simulink model "WindTurbine_System"  (R2023b)
settings: Solver=FixedStepAuto  StartTime=0.0  StopTime=24  FixedStep=1e-6  MaxStep=1e-6  RelTol=1e-3
values from neighbouring files (symbols this model uses):
  c1 = 0.22    [SystemParams.m]    (also in WindTurbineScript.m)
  c2 = 116    [SystemParams.m]    (also in WindTurbineScript.m)
  c3 = 0.4    [SystemParams.m]    (also in WindTurbineScript.m)
  c5 = 5    [SystemParams.m]    (also in WindTurbineScript.m)
  c6 = 12.5    [SystemParams.m]    (also in WindTurbineScript.m)
  C_boost = 50e-6    (= 5e-05)    [SystemParams.m]
  C_buck = 5e-6    (= 5e-06)    [SystemParams.m]
  C_rectifier = 1e-3    (= 0.001)    [SystemParams.m]
  Cp_sys = (Nr_cells_parallel * Cp_cell) / Nr_cells_series    [SystemParams.m]    (also in baterie.m)
  J = 0.8e-3    (= 0.0008)    [SystemParams.m]
  Ke = 0.175    [SystemParams.m]
  L_boost = 200e-6    (= 0.0002)    [SystemParams.m]
  L_buck = 300e-6    (= 0.0003)    [SystemParams.m]
  lambda_opt = 6.33    [SystemParams.m]    (also in WindTurbineScript.m)
  Ld = 1.53e-3    (= 0.00153)    [SystemParams.m]
  Lq = 1.53e-3    (= 0.00153)    [SystemParams.m]
  n1 = 15    [SystemParams.m]
  n2 = 1000    [SystemParams.m]
  omega_r = lambda_opt * wind_speed / R    (= 15.192)    [SystemParams.m]    (also in WindTurbineScript.m = omega_r_values(i))
  p = 4    [SystemParams.m]
  P_buck_v = 1.0e+03 * [0.01, 0.0427, 0.0854, 0.1282, 0.1709, 0.2136, 0.2563, 0.2990, 0.3418, 0.3845, 0.4272,                        0.4699, 0.5126, 0.5554, 0.5981, 0.6408, 0.6835, 0.7262, 0.7690, 0.8117, 0.8544,                        0.8971, 0.9398, 0.9826, 1.0253, 1.0680, 1.1107, 1.1534, 1.1962, 1.2389, 1.2816,                        1.3243, 1.3670, 1.4098, 1.4525, 1.4952, 1.5379, 1.5806, 1.6234, 1.6661, 1. ...(+623 chars)    [SystemParams.m]
  P_rec_v = 1.0e+03 * [0.01, 0.0432, 0.0864, 0.1296, 0.1727, 0.2159, 0.2591, 0.3023, 0.3455, 0.3887, 0.4319,                      0.4750, 0.5182, 0.5614, 0.6046, 0.6478, 0.6910, 0.7342, 0.7773, 0.8205, 0.8637,                      0.9069, 0.9501, 0.9933, 1.0365, 1.0796, 1.1228, 1.1660, 1.2092, 1.2524, 1.2956,                      1.3388, 1.3820, 1.4251, 1.4683, 1.5115, 1.5547, 1.5979, 1.6411, 1.6843, 1.7274,  ...(+605 chars)    [SystemParams.m]
  R = 5    [SystemParams.m]    (also in WindTurbineScript.m)
  R_buck_load_v = [230.4000, 53.9326, 26.9663, 17.9775, 13.4831, 10.7865, 8.9888, 7.7047, 6.7416, 5.9925, 5.3933,                   4.9030, 4.4944, 4.1487, 3.8523, 3.5955, 3.3708, 3.1725, 2.9963, 2.8386, 2.6966, 2.5682,                   2.4515, 2.3449, 2.2472, 2.1573, 2.0743, 1.9975, 1.9262, 1.8597, 1.7978, 1.7398, 1.6854,                   1.6343, 1.5863, 1.5409, 1.4981, 1.4576, 1.4193, 1.3829, 1.3483, 1.3154, 1. ...(+577 chars)    [SystemParams.m]
  R_rec_load_v = 1.0e+03 * [4.8400, 1.1204, 0.5602, 0.3735, 0.2803, 0.2242, 0.1868, 0.1601, 0.1401, 0.1245, 0.1121,                            0.1019, 0.0934, 0.0862, 0.0801, 0.0747, 0.0700, 0.0659, 0.0623, 0.0590, 0.0560, 0.0534,                            0.0509, 0.0487, 0.0467, 0.0448, 0.0431, 0.0415, 0.0400, 0.0386, 0.0374, 0.0362, 0.0350,                            0.0340, 0.0330, 0.0320, 0.0311, 0.0303, 0.02 ...(+634 chars)    [SystemParams.m]
  ro = 1.225    [SystemParams.m]    (also in WindTurbineScript.m)
  Rp_sys = (Nr_cells_series * Rp_cell) / Nr_cells_parallel    [SystemParams.m]    (also in baterie.m)
  Rs = 2.875    [SystemParams.m]    (also in VOC_1C_3pulse_14rest.mat = 0.09415625)
  Rs_sys = (Nr_cells_series * Rs_cell) / Nr_cells_parallel    [SystemParams.m]    (also in baterie.m)
  State_Of_Charge = 65    [SystemParams.m]
libraries: simulink x4, slpidlib x2, SignalEditorBlockLib x1
(part 1 of 2)
settings Model: SimulationMode=accelerator  Creator=tudorn  LastModifiedBy=tudorn
settings HardwareCC: ProdBitPerLong=64  ProdHWDeviceType=Apple->ARM64

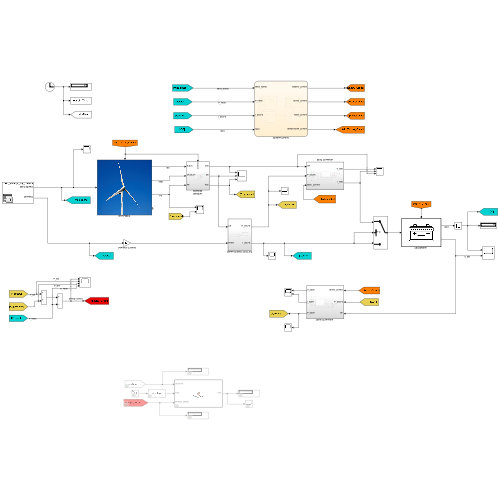
[thumbnail: Simulink's stored preview of the top-level diagram]
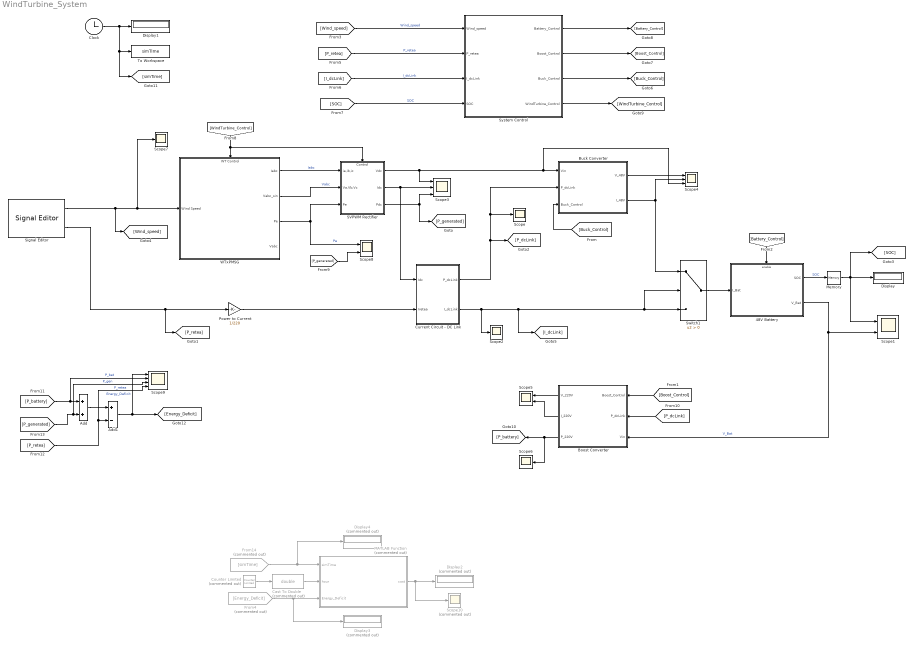
== system WindTurbine_System ==
  "48V Battery " : Subsystem
      mask Display: image('batteryPhoto.png');
  Add : Sum
  Add1 : Sum  Inputs=+-
  Boost Converter : Subsystem
  Buck Converter : Subsystem
  Cast To Double : DataTypeConversion  Commented=on  OutDataTypeStr=double  SaturateOnIntegerOverflow=off  RndMeth=Floor
  Clock : Clock
  Counter Limited : simulink/Sources/Counter Limited  Commented=on  uplimit=24  tsamp=1
  Current Circuit - DC Link : Subsystem
  Display : Display
  Display1 : Display
  Display2 : Display  Commented=on
  Display3 : Display  Commented=on
  Display4 : Display  Commented=on
  From14 : From  Commented=on  GotoTag=simTime
  From4 : From  Commented=on  GotoTag=Energy_Deficit
  MATLAB Function : MATLAB Function  Commented=on  TreatAsAtomicUnit=on
  Memory : Memory  InitialCondition=State_Of_Charge
  Power to Current : Gain  Gain=1/220
  SVPWM Rectifier : Subsystem
      settings: PortSchema="{\"entries\":[{\"content\":{\"sides\":[{\"content\":{\"connectorIds\":[\"In1\",\"In2\",\"In3\"]},\"type\":\"ConnectorPlacement.EquallySpacedRectSide\",\"uuid\":\"47eca95a-203c-4150-b63f-06b4ee16708d\"},{\"content\":{\"connectorIds\":[\"Out1\",\"Out2\",\"Out3\"],\"side\":\"RIGHT\"},\"type\":\"ConnectorPlacement.EquallySpacedRectSide\",\"uuid\":\"e6ad715a-a702-4d71-ac1c-337baa4d9820\"},{\"content\":{\"connectorIds\":[\"In4\"],\"side\":\"TOP\"},\"type\":\"ConnectorPlacement.EquallySpacedRectSide\",\"uuid\":\"da1a96bd-35b5-4cd5-85b2-7e6a1b4649ba\"}]},\"type\":\"ConnectorPlacement.EquallySpacedConnector\",\"uuid\":\"95ca3103-3ae0-40eb-bfd8-7b543be5b023\"}],\"packageUris\":[\"http://schema.mathworks.com/mf0/Connector/R2020b\"],\"version\":\"1.0\"}"
  Scope{,2,6..7} (4 alike) : Scope
  Scope1 : Scope  NumInputPorts=2
  Scope10 : Scope  Commented=on
  Scope3 : Scope  NumInputPorts=3
  Scope4 : Scope  NumInputPorts=3
  Scope5 : Scope  NumInputPorts=2
  Scope8 : Scope  NumInputPorts=2
  Scope9 : Scope  NumInputPorts=4
  Signal Editor : SignalEditorBlockLib/Signal Editor  FileName=ConstWind_VarDemand.mat  ActiveScenario=x24h_Increase_WS_Demand  ActiveSignal=Wind Speed  IsBus=off  OutputBusObjectStr=Bus: BusObject  SampleTime=0  Interpolate=off  ZeroCross=off  OutputAfterFinalValue=Setting to zero  Unit=inherit  PreserveSignalName=on  ApplySigPropsToAllScenarios=on  ApplySigPropsToAllSignals=off
  Switch1 : Switch  Criteria=u2 > Threshold  SaturateOnIntegerOverflow=off  InputSameDT=off
  System Control : Stateflow chart  TreatAsAtomicUnit=on
  To Workspace : ToWorkspace  VariableName=simTIme  SaveFormat=Timeseries  SampleTime=-1
  WTxPMSG : Subsystem
      settings: PortSchema="{\"entries\":[{\"content\":{\"sides\":[{\"content\":{\"connectorIds\":[\"In1\"]},\"type\":\"ConnectorPlacement.EquallySpacedRectSide\",\"uuid\":\"6e920366-051d-4787-8dda-26163d9164f0\"},{\"content\":{\"connectorIds\":[\"Out1\",\"Out2\",\"Out3\",\"Out4\"],\"side\":\"RIGHT\"},\"type\":\"ConnectorPlacement.EquallySpacedRectSide\",\"uuid\":\"50211027-c95a-4b04-b652-faaace106a3a\"},{\"content\":{\"connectorIds\":[\"In2\"],\"side\":\"TOP\"},\"type\":\"ConnectorPlacement.EquallySpacedRectSide\",\"uuid\":\"d93d5085-7e12-4e15-83b4-3ac4d8b1a417\"}]},\"type\":\"ConnectorPlacement.EquallySpacedConnector\",\"uuid\":\"325f5742-bcf0-41bb-9a35-ab4334df2944\"}],\"packageUris\":[\"http://schema.mathworks.com/mf0/Connector/R2020b\"],\"version\":\"1.0\"}"
      mask Display: image('windTurbinePhoto.png');
  wires:
  [P_generated] -> Scope9/3, Add/2  "P_gen"
  WTxPMSG/3(Pe) -> SVPWM Rectifier/3(Pe), Scope8/1  "Pe"
  "48V Battery "/2(V_Bat) -> Boost Converter/3(Vin), Scope1/2  "V_Bat"
  [Buck_Control] -> Buck Converter/3(Buck_Control)
  [WindTurbine_Control] -> SVPWM Rectifier/4(Control), WTxPMSG/2(WT Control)
  Current Circuit - DC Link/2(I_dcLink) -> Scope2/1, [I_dcLink], Switch1/2, Switch1/3
  Current Circuit - DC Link/1(P_dcLink) -> [P_dcLink], Scope/1, Buck Converter/2(P_dcLink)
  [P_battery] -> Scope9/2, Add/1  "P_bat"
  Boost Converter/1(V_220V) -> Scope5/1
  Add/1 -> Add1/1
  Power to Current/1 -> Current Circuit - DC Link/2(Iretea)
  WTxPMSG/2(Vabc_sin) -> SVPWM Rectifier/2(Va,Vb,Vc)  "Vabc"
  Switch1/1 -> "48V Battery "/1(I_Bat)
  "48V Battery "/1(SOC) -> Memory/1  "SOC"
  Buck Converter/2(I_48V) -> Scope4/2, Switch1/1
  SVPWM Rectifier/3(Pdc) -> Scope3/3, [P_generated]
  [Battery_Control] -> "48V Battery "/Enable
  Buck Converter/1(V_48V) -> Scope4/1
  [P_dcLink] -> Boost Converter/2(P_dcLink)
  Memory/1 -> [SOC], Display/1, Scope1/1
  [P_generated] -> Scope8/2
  SVPWM Rectifier/1(Vdc) -> Scope4/3, Buck Converter/1(Vin), Scope3/1
  WTxPMSG/1(Iabc) -> SVPWM Rectifier/1(ia,ib,ic)  "Iabc"
  Signal Editor/1 -> Scope7/1, WTxPMSG/1(Wind Speed), [Wind_speed]
  Signal Editor/2 -> Power to Current/1, [P_retea]
  Clock/1 -> [simTime], To Workspace/1, Display1/1
  [P_retea] -> Scope9/4, Add1/2  "P_retea"
  Boost Converter/2(I_220V) -> Scope5/2
  Add1/1 -> Scope9/1, [Energy_Deficit]  "Energy_Deficit"
  [Boost_Control] -> Boost Converter/1(Boost_Control)
  Boost Converter/3(P_220V) -> [P_battery], Scope6/1
  SVPWM Rectifier/2(Idc) -> Scope3/2, Current Circuit - DC Link/1(Idc)
  [P_retea] -> System Control/2(P_retea)  "P_retea"
  [Wind_speed] -> System Control/1(Wind_speed)  "Wind_speed"
  System Control/3(Buck_Control) -> [Buck_Control]
  [I_dcLink] -> System Control/3(I_dcLink)  "I_dcLink"
  System Control/4(WindTurbine_Control) -> [WindTurbine_Control]
  [SOC] -> System Control/4(SOC)  "SOC"
  System Control/2(Boost_Control) -> [Boost_Control]
  System Control/1(Battery_Control) -> [Battery_Control]
  MATLAB Function/1(cost) -> Scope10/1, Display2/1
  From4/1 -> Display3/1, MATLAB Function/3(Energy_Deficit)
  From14/1 -> Display4/1, MATLAB Function/1(simTime)
  Counter Limited/1 -> Cast To Double/1
  Cast To Double/1 -> MATLAB Function/2(hour)

== system WindTurbine_System/48V Battery  ==
  I_Bat : Inport
  Enable : EnablePort
  (14 - 96)% SOC : Saturate  UpperLimit=96  LowerLimit=14
  Add : Sum  Inputs=+++
  Cp : Constant  Value=Cp_sys
  RC Network : Subsystem
  Rp : Constant  Value=Rp_sys
  Rs : Gain  Gain=Rs_sys
  SOC Calculation1 : Subsystem
  SOC_OCV : Subsystem
  Saturation : Saturate  UpperLimit=93.75  LowerLimit=-93.75
  Scope : Scope
  Scope1 : Scope
  Scope2 : Scope
  SOC : Outport
  V_Bat : Outport  Port=2
  wires:
  RC Network/1(V1) -> Scope2/1, Add/2
  SOC_OCV/1(OCV) -> Add/1
  Rp/1 -> RC Network/2(Rp)
  Cp/1 -> RC Network/3(Cp)
  Rs/1 -> Add/3  "Vs - Voltage drop on the Series Resistance"
  Add/1 -> Scope1/1, V_Bat/1
  SOC Calculation1/1(SOC) -> (14 - 96)% SOC/1
  (14 - 96)% SOC/1 -> Scope/1, SOC/1, SOC_OCV/1(SOC)
  I_Bat/1 -> Saturation/1
  Saturation/1 -> SOC Calculation1/1(I_Bat), Rs/1, RC Network/1(I_Bat)

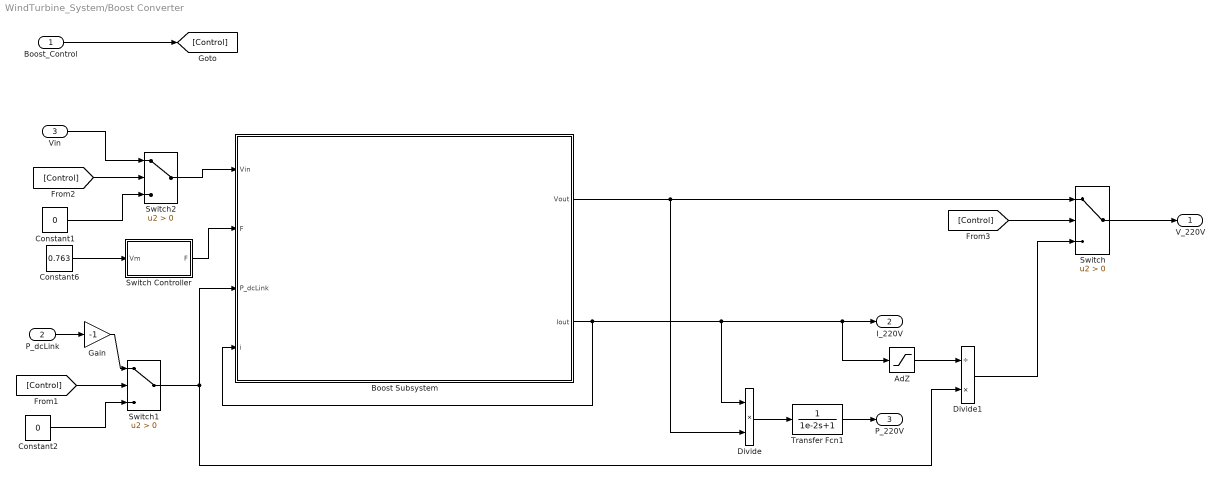
== system WindTurbine_System/Boost Converter ==
  Boost_Control : Inport
  P_dcLink : Inport  Port=2
  Vin : Inport  Port=3
  AdZ : Saturate  UpperLimit=inf  LowerLimit=1e-6
  Boost Subsystem : Subsystem
  Constant1 : Constant  Value=0
  Constant2 : Constant  Value=0
  Constant6 : Constant  Value=0.763
  Divide : Product  Inputs=**
  Divide1 : Product  Inputs=/*
  Gain : Gain  Gain=-1
  Switch : Switch  Criteria=u2 > Threshold  SaturateOnIntegerOverflow=off  InputSameDT=off
  Switch Controller : Subsystem
  Switch1 : Switch  Criteria=u2 > Threshold  SaturateOnIntegerOverflow=off  InputSameDT=off
  Switch2 : Switch  Criteria=u2 > Threshold  SaturateOnIntegerOverflow=off  InputSameDT=off
  Transfer Fcn1 : TransferFcn  Denominator=[1e-2 1]
  V_220V : Outport
  I_220V : Outport  Port=2
  P_220V : Outport  Port=3
  wires:
  Constant6/1 -> Switch Controller/1(Vm)
  Switch Controller/1(F) -> Boost Subsystem/2(F)
  Divide/1 -> Transfer Fcn1/1
  Transfer Fcn1/1 -> P_220V/1
  Boost Subsystem/1(Vout) -> Switch/1, Divide/2
  Boost Subsystem/2(Iout) -> Divide/1, AdZ/1, I_220V/1, Boost Subsystem/4(i)
  Boost_Control/1 -> [Control]
  Constant1/1 -> Switch2/3
  [Control] -> Switch2/2
  Switch2/1 -> Boost Subsystem/1(Vin)
  Vin/1 -> Switch2/1
  Constant2/1 -> Switch1/3
  [Control] -> Switch1/2
  P_dcLink/1 -> Gain/1
  Gain/1 -> Switch1/1
  Switch1/1 -> Divide1/2, Boost Subsystem/3(P_dcLink)
  [Control] -> Switch/2
  Switch/1 -> V_220V/1
  Divide1/1 -> Switch/3
  AdZ/1 -> Divide1/1

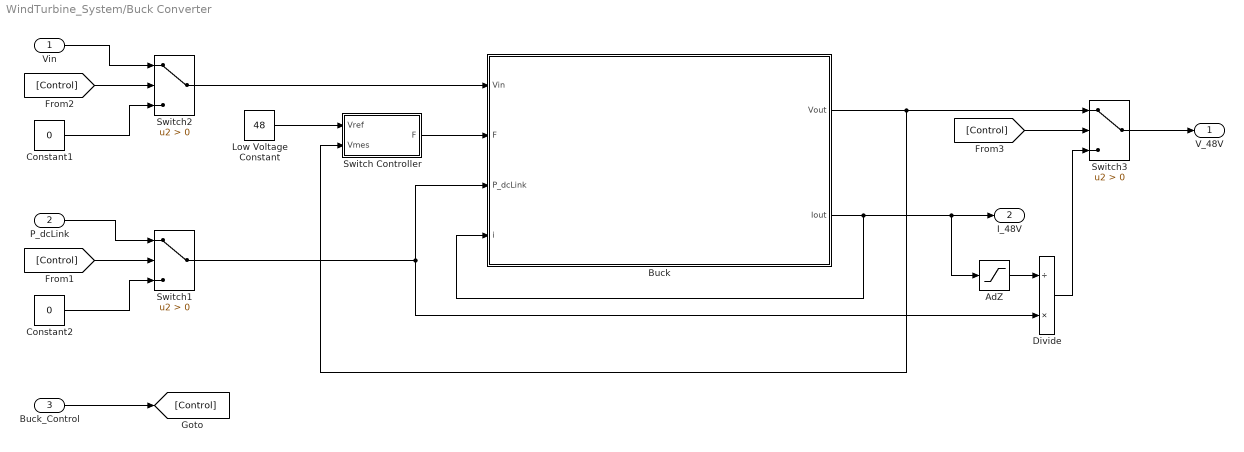
== system WindTurbine_System/Buck Converter ==
  Vin : Inport
  P_dcLink : Inport  Port=2
  Buck_Control : Inport  Port=3
  AdZ : Saturate  UpperLimit=inf  LowerLimit=1e-6
  Buck : Subsystem
  Constant1 : Constant  Value=0
  Constant2 : Constant  Value=0
  Divide : Product  Inputs=/*
  Low Voltage Constant : Constant  Value=48
  Switch Controller : Subsystem
  Switch1 : Switch  Criteria=u2 > Threshold  SaturateOnIntegerOverflow=off  InputSameDT=off
  Switch2 : Switch  Criteria=u2 > Threshold  SaturateOnIntegerOverflow=off  InputSameDT=off
  Switch3 : Switch  Criteria=u2 > Threshold  SaturateOnIntegerOverflow=off  InputSameDT=off
  V_48V : Outport
  I_48V : Outport  Port=2
  wires:
  Low Voltage Constant/1 -> Switch Controller/1(Vref)
  Switch Controller/1(F) -> Buck/2(F)
  Buck/1(Vout) -> Switch Controller/2(Vmes), Switch3/1
  Buck/2(Iout) -> AdZ/1, I_48V/1, Buck/4(i)
  Buck_Control/1 -> [Control]
  [Control] -> Switch2/2
  Constant1/1 -> Switch2/3
  Switch2/1 -> Buck/1(Vin)
  Vin/1 -> Switch2/1
  Constant2/1 -> Switch1/3
  [Control] -> Switch1/2
  Switch1/1 -> Divide/2, Buck/3(P_dcLink)
  P_dcLink/1 -> Switch1/1
  Switch3/1 -> V_48V/1
  [Control] -> Switch3/2
  Divide/1 -> Switch3/3
  AdZ/1 -> Divide/1

== system WindTurbine_System/Current Circuit - DC Link ==
  Idc : Inport
  Iretea : Inport  Port=2
  Add : Sum  Inputs=+-
  Gain : Gain  Gain=220
  P_dcLink : Outport
  I_dcLink : Outport  Port=2
  wires:
  Idc/1 -> Add/1
  Iretea/1 -> Add/2
  Add/1 -> Gain/1, I_dcLink/1
  Gain/1 -> P_dcLink/1

== system WindTurbine_System/SVPWM Rectifier ==
  ia,ib,ic : Inport
  Va,Vb,Vc : Inport  Port=2
  Pe : Inport  Port=3
  Control : Inport  Port=4
  AdZ : Saturate  UpperLimit=inf  LowerLimit=1e-6
  Divide : Product  Inputs=**
  Divide1 : Product  Inputs=/*
  Saturation : Saturate  UpperLimit=220  LowerLimit=0
  Space Vector PWM : Subsystem
  Switch : Switch  Criteria=u2 > Threshold  SaturateOnIntegerOverflow=off  InputSameDT=off
  V_DC Calculation : Subsystem
  Vdc : Outport
  Idc : Outport  Port=2
  Pdc : Outport  Port=3
  wires:
  Va,Vb,Vc/1 -> Space Vector PWM/1("Va, Vb, Vc")
  V_DC Calculation/2(Idc) -> AdZ/1, Idc/1, Divide/1
  ia,ib,ic/1 -> V_DC Calculation/1("Ia, Ib, Ic")
  Space Vector PWM/1(Sa,Sb,Sc) -> V_DC Calculation/2("Sa, Sb, Sc")
  Pe/1 -> V_DC Calculation/3(Pe), Divide1/2
  Switch/1 -> Vdc/1
  Control/1 -> Switch/2
  V_DC Calculation/1(Vdc) -> Switch/1, Divide/2
  Divide1/1 -> Saturation/1
  Divide/1 -> Pdc/1
  AdZ/1 -> Divide1/1
  Saturation/1 -> Switch/3

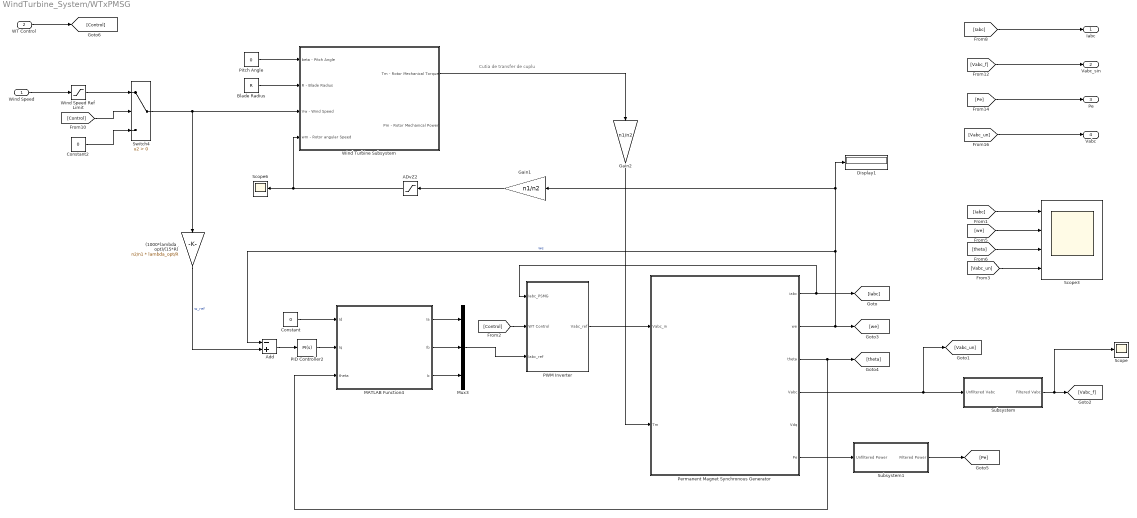
== system WindTurbine_System/WTxPMSG ==
  note: Cutia de transfer de cuplu
  Wind Speed : Inport
  WT Control : Inport  Port=2
  (1000*lambda_opt)/(15*R) : Gain  Gain=n2/n1 * lambda_opt/R
  ADvZ2 : Saturate  UpperLimit=omega_r  LowerLimit=1e-6
  Add : Sum  Inputs=-+
  Blade Radius : Constant  Value=R
  Constant : Constant  Value=0
  Constant2 : Constant  Value=0
  Display1 : Display
  Gain1 : Gain  Gain=n1/n2
  Gain2 : Gain  Gain=n1/n2
  MATLAB Function4 : MATLAB Function  TreatAsAtomicUnit=on
  Mux3 : Mux  Inputs=3
  PID Controller2 : slpidlib/PID Controller  Controller=PI  Form=Parallel  TimeDomain=Continuous-time  UseExternalTs=off  SampleTime=-1  IntegratorMethod=Forward Euler  FilterMethod=Forward Euler  ControllerParametersSource=internal  P=40  I=3  UseKiTs=off  D=0  N=100  UseFilter=on  TunerSelectOption=Transfer Function Based (PID Tuner App)  InitialConditionSource=internal  InitialConditionForIntegrator=0  InitialConditionForFilter=0  DifferentiatorICPrevScaledInput=0  ExternalReset=none  TrackingMode=off  Kt=1  LimitOutput=off  SatLimitsSource=internal  UpperSaturationLimit=inf  LowerSaturationLimit=-inf  LinearizeAsGain=on  AntiWindupMode=none  Kb=1  LimitIntegrator=off  UpperIntegratorSaturationLimit=inf  LowerIntegratorSaturationLimit=-inf  POutMin=[]  POutMax=[]  IOutMin=[]  IOutMax=[]  DOutMin=[]  DOutMax=[]  NOutMin=[]  NOutMax=[]  SumOutMin=[]  SumOutMax=[]  SaturationOutMin=[]  SaturationOutMax=[]  PParamMin=[]  PParamMax=[]  IParamMin=[]  IParamMax=[]  DParamMin=[]  DParamMax=[]  NParamMin=[]  NParamMax=[]  KbParamMin=[]  KbParamMax=[]  KtParamMin=[]  KtParamMax=[]  KbOutMin=[]  KbOutMax=[]  KtOutMin=[]  KtOutMax=[]  IntegratorOutMin=[]  IntegratorOutMax=[]  FilterOutMin=[]  FilterOutMax=[]  SumI1OutMin=[]  SumI1OutMax=[]  SumI2OutMin=[]  SumI2OutMax=[]  SumI3OutMin=[]  SumI3OutMax=[]  SumI4OutMin=[]  SumI4OutMax=[]  SumDOutMin=[]  SumDOutMax=[]  DifferentiatorOutMin=[]  DifferentiatorOutMax=[]  FilterDiffOutCoefMin=[]  FilterDiffOutCoefMax=[]  ReciprocalOutMin=[]  ReciprocalOutMax=[]  SumDenOutMin=[]  SumDenOutMax=[]  SumNumOutMin=[]  SumNumOutMax=[]  DivideOutMin=[]  DivideOutMax=[]  UdiffTsProdOutMin=[]  UdiffTsProdOutMax=[]  NTsProdOutMin=[]  NTsProdOutMax=[]  UintegralTsProdOutMin=[]  UintegralTsProdOutMax=[]  UngainTsProdOutMin=[]  UngainTsProdOutMax=[]  ClampingZeroOutDataTypeStr=Inherit: Inherit via back propagation  ClampingZeroOutMin=[]  ClampingZeroOutMax=[]  FilterDenConstantOutDataTypeStr=Inherit: Inherit via back propagation  FilterDenConstantOutMin=[]  FilterDenConstantOutMax=[]  PCopyOutDataTypeStr=Inherit: Inherit via back propagation  PCopyOutMin=[]  PCopyOutMax=[]  NCopyOutDataTypeStr=Inherit: Inherit via back propagation  NCopyOutMin=[]  NCopyOutMax=[]  IntegratorContinuousStateAttributes=''  IntegratorStateMustResolveToSignalObject=off  IntegratorRTWStateStorageClass=Auto  FilterContinuousStateAttributes=''  FilterStateMustResolveToSignalObject=off  FilterRTWStateStorageClass=Auto  ParallelPVariant=InternalParameters  IdealPVariant=Disabled  IVariant=InternalParameters  DVariant=Disabled  IntegratorVariant=Continuous  SatVariant=Disabled  AWVariant=Passthrough  PCopyVariant=Disabled  TRVariant=Disabled  FdbkBlocksVariant=Forward  IdealPFdbkVariant=Disabled  SatFdbkVariant=Disabled  DerivativeFilterVariant=Disabled  NVariant=Disabled  NCopyVariant=Disabled_SignalSpec  FilterICVariant=Disabled  IntegratorICVariant=InternalICs  ExternalResetVariant=Disabled  TRSumVariant=Passthrough  SumFdbkVariant=Disabled  SumVariant=Sum_PI  TsampFilterVariant=InternalTs  TsampNgainVariant=Passthrough  TsampIntegralVariant=Disabled_SignalSpec  ExternalSaturationOutDataTypeStr=Inherit: Same as second input
  PWM Inverter : Subsystem
  Permanent Magnet Synchronous Generator : Subsystem
  Pitch Angle : Constant  Value=0
  Scope : Scope
  Scope3 : Scope  NumInputPorts=4
  Scope6 : Scope
  Subsystem : Subsystem
  Subsystem1 : Subsystem
  Switch4 : Switch  Criteria=u2 > Threshold  SaturateOnIntegerOverflow=off  InputSameDT=off
  Wind Speed Ref Limit : Saturate  UpperLimit=12  LowerLimit=0
  Wind Turbine Subsystem : Subsystem
  Iabc : Outport
  Vabc_sin : Outport  Port=2
  Pe : Outport  Port=3
  Vabc : Outport  Port=4
  wires:
  Pitch Angle/1 -> Wind Turbine Subsystem/1(beta - Pitch Angle)
  Gain1/1 -> ADvZ2/1
  Add/1 -> PID Controller2/1
  MATLAB Function4/1(Ia) -> Mux3/1
  Permanent Magnet Synchronous Generator/3(theta) -> [theta], MATLAB Function4/3(theta)
  Constant/1 -> MATLAB Function4/1(Id)
  Blade Radius/1 -> Wind Turbine Subsystem/2(R - Blade Radius)
  PID Controller2/1 -> MATLAB Function4/2(Iq)
  Mux3/1 -> PWM Inverter/3(Iabc_ref)
  Permanent Magnet Synchronous Generator/4(Vabc) -> Subsystem/1(Unfiltered Vabc), [Vabc_un]
  Permanent Magnet Synchronous Generator/1(iabc) -> PWM Inverter/1(Iabc_PSMG), [Iabc]
  MATLAB Function4/2(Ib) -> Mux3/2
  (1000*lambda_opt)/(15*R)/1 -> Add/2  "w_ref"
  PWM Inverter/1(Vabc_ref) -> Permanent Magnet Synchronous Generator/1(Vabc_in)
  Wind Speed/1 -> Wind Speed Ref Limit/1
  MATLAB Function4/3(Ic) -> Mux3/3
  ADvZ2/1 -> Scope6/1, Wind Turbine Subsystem/4(wm - Rotor angular Speed)
  Permanent Magnet Synchronous Generator/2(we) -> [we], Display1/1, Gain1/1, Add/1  "we"
  Gain2/1 -> Permanent Magnet Synchronous Generator/2(Tm)
  Wind Turbine Subsystem/1(Tm - Rotor Mechanical Torque) -> Gain2/1
  [Iabc] -> Scope3/1
  Subsystem/1(Filtered Vabc) -> Scope/1, [Vabc_f]
  [Vabc_un] -> Scope3/4
  Permanent Magnet Synchronous Generator/6(Pe) -> Subsystem1/1(Unfiltered Power)
  [we] -> Scope3/2
  [theta] -> Scope3/3
  Subsystem1/1(Filtered Power) -> [Pe]
  WT Control/1 -> [Control]
  [Control] -> Switch4/2
  Wind Speed Ref Limit/1 -> Switch4/1
  Switch4/1 -> (1000*lambda_opt)/(15*R)/1, Wind Turbine Subsystem/3(Vw - Wind Speed)
  Constant2/1 -> Switch4/3
  [Iabc] -> Iabc/1
  [Vabc_f] -> Vabc_sin/1
  [Pe] -> Pe/1
  [Vabc_un] -> Vabc/1
  [Control] -> PWM Inverter/2(WT Control)

== system WindTurbine_System/48V Battery /RC Network ==
  I_Bat : Inport
  Rp : Inport  Port=2
  Cp : Inport  Port=3
  Add : Sum  Inputs=+-
  Divide : Product  Inputs=/*
  Divide1 : Product  Inputs=**
  Divide2 : Product  Inputs=*/
  Integrator : Integrator
  Scope : Scope
  Scope1 : Scope
  V1 : Outport
  wires:
  Cp/1 -> Divide2/2, Divide1/1
  Rp/1 -> Divide1/2
  I_Bat/1 -> Divide2/1
  Divide2/1 -> Add/1  "I/Cp"
  Add/1 -> Scope/1, Integrator/1  "V1dot"
  Divide/1 -> Add/2  "V1/(Cp*Rp)"
  Divide1/1 -> Divide/1
  Integrator/1 -> Scope1/1, V1/1, Divide/2

== system WindTurbine_System/48V Battery /SOC Calculation1 ==
  I_Bat : Inport
  "Ah -> As" : Gain  Gain=1/36
  Battery Cap (Ah) : Constant  Value=1111
  Display : Display
  Display1 : Display
  Divide2 : Product  Inputs=*/
  SOC0 : Integrator  InitialCondition=State_Of_Charge
  SOC : Outport
  wires:
  SOC0/1 -> Display1/1, SOC/1
  Divide2/1 -> Display/1, SOC0/1  "I_Bat/Cap_Bat"
  I_Bat/1 -> "Ah -> As"/1
  Battery Cap (Ah)/1 -> Divide2/2
  "Ah -> As"/1 -> Divide2/1

== system WindTurbine_System/48V Battery /SOC_OCV ==
  SOC : Inport
  1-D Lookup Table : Lookup_n-D  NumberOfTableDimensions=1  BreakpointsForDimension1=[0 5 9.5 14 20 30 40 50 60 70 80 90 96 99 99.5 100]  Table=[40, 44.8, 48, 50.40, 51.20, 51.60, 52, 52.20, 52.40, 52.80, 53.20, 53.60, 52.80, 54, 55.20, 58.40]  InternalRulePriority=Speed  RndMeth=Simplest
  OCV : Outport
  wires:
  SOC/1 -> 1-D Lookup Table/1
  1-D Lookup Table/1 -> OCV/1

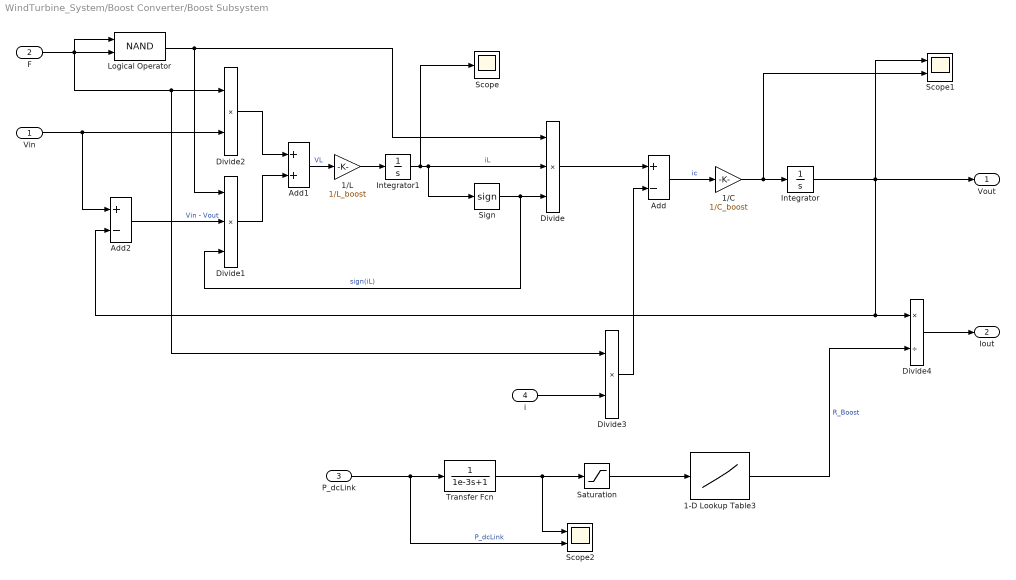
== system WindTurbine_System/Boost Converter/Boost Subsystem ==
  Vin : Inport
  F : Inport  Port=2
  P_dcLink : Inport  Port=3
  i : Inport  Port=4
  1-D Lookup Table3 : Lookup_n-D  NumberOfTableDimensions=1  BreakpointsForDimension1=P_rec_v  Table=R_rec_load_v  InternalRulePriority=Speed  RndMeth=Simplest
  1/C : Gain  Gain=1/C_boost
  1/L : Gain  Gain=1/L_boost
  Add : Sum  Inputs=+-
  Add1 : Sum
  Add2 : Sum  Inputs=+-
  Divide : Product  Inputs=***
  Divide1 : Product  Inputs=***
  Divide2 : Product  Inputs=**
  Divide3 : Product  Inputs=**
  Divide4 : Product  Inputs=*/
  Integrator : Integrator  LimitOutput=on  UpperSaturationLimit=220  LowerSaturationLimit=-220
  Integrator1 : Integrator
  Logical Operator : Logic  Operator=NAND  AllPortsSameDT=off  OutDataTypeStr=boolean
  Saturation : Saturate  UpperLimit=inf  LowerLimit=1
  Scope : Scope
  Scope1 : Scope  NumInputPorts=2
  Scope2 : Scope  NumInputPorts=2
  Sign : Signum  ZeroCross=off
  Transfer Fcn : TransferFcn  Denominator=[1e-3 1]
  Vout : Outport
  Iout : Outport  Port=2
  wires:
  Add/1 -> 1/C/1  "ic"
  Divide/1 -> Add/1
  Sign/1 -> Divide1/3, Divide/3  "sign(iL)"
  1/L/1 -> Integrator1/1
  Integrator1/1 -> Scope/1, Sign/1, Divide/2  "iL"
  Vin/1 -> Add2/1, Divide2/2
  Add2/1 -> Divide1/2  "Vin - Vout"
  F/1 -> Divide2/1, Divide3/1, Logical Operator/1, Logical Operator/2
  Logical Operator/1 -> Divide/1, Divide1/1
  Add1/1 -> 1/L/1  "VL"
  Divide2/1 -> Add1/1
  Divide1/1 -> Add1/2
  Divide4/1 -> Iout/1
  i/1 -> Divide3/2
  Divide3/1 -> Add/2
  1-D Lookup Table3/1 -> Divide4/2  "R_Boost"
  Saturation/1 -> 1-D Lookup Table3/1
  P_dcLink/1 -> Scope2/2, Transfer Fcn/1  "P_dcLink"
  Transfer Fcn/1 -> Scope2/1, Saturation/1
  1/C/1 -> Scope1/2, Integrator/1
  Integrator/1 -> Scope1/1, Add2/2, Divide4/1, Vout/1

== system WindTurbine_System/Boost Converter/Switch Controller ==
  Vm : Inport
  Relational Operator1 : RelationalOperator  Operator=>  OutDataTypeStr=boolean  RndMeth=Simplest  InputSameDT=off
  Repeating Sequence1 : simulink/Sources/Repeating Sequence  rep_seq_t=[0 0.5 1]/50e3  rep_seq_y=[0 1 0]
  F : Outport
  wires:
  Repeating Sequence1/1 -> Relational Operator1/2
  Relational Operator1/1 -> F/1
  Vm/1 -> Relational Operator1/1

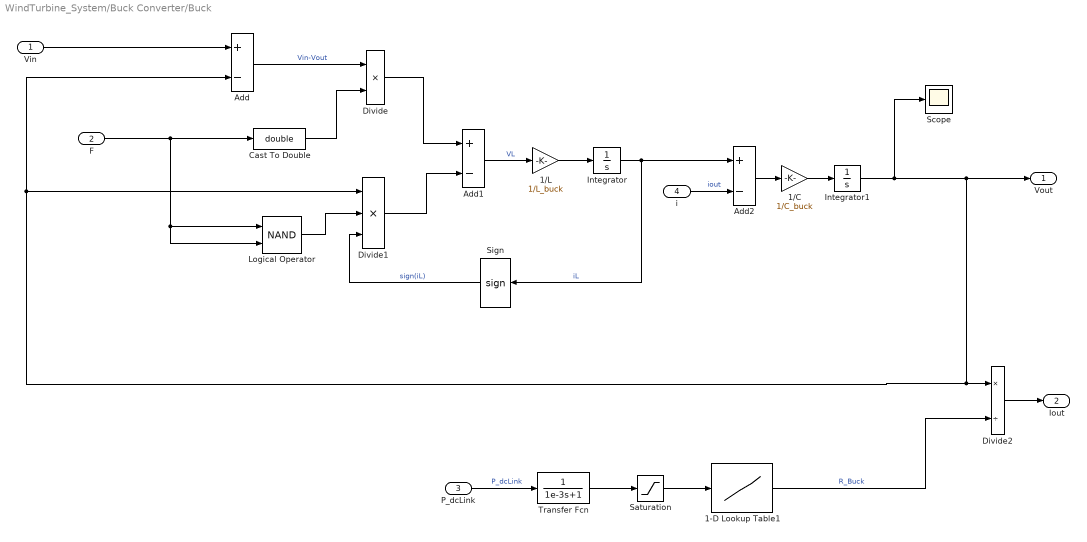
== system WindTurbine_System/Buck Converter/Buck ==
  Vin : Inport
  F : Inport  Port=2
  P_dcLink : Inport  Port=3
  i : Inport  Port=4
  1-D Lookup Table1 : Lookup_n-D  NumberOfTableDimensions=1  BreakpointsForDimension1=P_buck_v  Table=R_buck_load_v  InternalRulePriority=Speed  RndMeth=Simplest
  1/C : Gain  Gain=1/C_buck
  1/L : Gain  Gain=1/L_buck
  Add : Sum  Inputs=+-
  Add1 : Sum  Inputs=+-
  Add2 : Sum  Inputs=+-
  Cast To Double : DataTypeConversion  OutDataTypeStr=double  SaturateOnIntegerOverflow=off  RndMeth=Floor
  Divide : Product  Inputs=**
  Divide1 : Product  Inputs=***
  Divide2 : Product  Inputs=*/
  Integrator : Integrator
  Integrator1 : Integrator  LimitOutput=on  UpperSaturationLimit=48  LowerSaturationLimit=-48
  Logical Operator : Logic  Operator=NAND  AllPortsSameDT=off  OutDataTypeStr=boolean
  Saturation : Saturate  UpperLimit=inf  LowerLimit=1
  Scope : Scope
  Sign : Signum  ZeroCross=off
  Transfer Fcn : TransferFcn  Denominator=[1e-3 1]
  Vout : Outport
  Iout : Outport  Port=2
  wires:
  Vin/1 -> Add/1
  Add/1 -> Divide/1  "Vin-Vout"
  Divide/1 -> Add1/1
  Divide1/1 -> Add1/2
  Add1/1 -> 1/L/1  "VL"
  1/L/1 -> Integrator/1
  Integrator/1 -> Add2/1, Sign/1  "iL"
  Add2/1 -> 1/C/1
  i/1 -> Add2/2  "iout"
  F/1 -> Logical Operator/2, Logical Operator/1, Cast To Double/1
  Sign/1 -> Divide1/3  "sign(iL)"
  Logical Operator/1 -> Divide1/2
  Cast To Double/1 -> Divide/2
  Divide2/1 -> Iout/1
  1-D Lookup Table1/1 -> Divide2/2  "R_Buck"
  P_dcLink/1 -> Transfer Fcn/1  "P_dcLink"
  Saturation/1 -> 1-D Lookup Table1/1
  Transfer Fcn/1 -> Saturation/1
  1/C/1 -> Integrator1/1
  Integrator1/1 -> Scope/1, Divide1/1, Add/2, Divide2/1, Vout/1

== system WindTurbine_System/Buck Converter/Switch Controller ==
  Vref : Inport
  Vmes : Inport  Port=2
  Add : Sum  Inputs=+-
  PID Controller1 : slpidlib/PID Controller  Controller=PI  Form=Parallel  TimeDomain=Continuous-time  UseExternalTs=off  SampleTime=-1  IntegratorMethod=Forward Euler  FilterMethod=Forward Euler  ControllerParametersSource=internal  P=0  I=13.2  UseKiTs=off  D=1.7e-5  N=100  UseFilter=on  TunerSelectOption=Transfer Function Based (PID Tuner App)  InitialConditionSource=internal  InitialConditionForIntegrator=0  InitialConditionForFilter=0  DifferentiatorICPrevScaledInput=0  ExternalReset=none  TrackingMode=off  Kt=1  LimitOutput=off  SatLimitsSource=internal  UpperSaturationLimit=inf  LowerSaturationLimit=-inf  LinearizeAsGain=on  AntiWindupMode=none  Kb=1  LimitIntegrator=off  UpperIntegratorSaturationLimit=inf  LowerIntegratorSaturationLimit=-inf  POutMin=[]  POutMax=[]  IOutMin=[]  IOutMax=[]  DOutMin=[]  DOutMax=[]  NOutMin=[]  NOutMax=[]  SumOutMin=[]  SumOutMax=[]  SaturationOutMin=[]  SaturationOutMax=[]  PParamMin=[]  PParamMax=[]  IParamMin=[]  IParamMax=[]  DParamMin=[]  DParamMax=[]  NParamMin=[]  NParamMax=[]  KbParamMin=[]  KbParamMax=[]  KtParamMin=[]  KtParamMax=[]  KbOutMin=[]  KbOutMax=[]  KtOutMin=[]  KtOutMax=[]  IntegratorOutMin=[]  IntegratorOutMax=[]  FilterOutMin=[]  FilterOutMax=[]  SumI1OutMin=[]  SumI1OutMax=[]  SumI2OutMin=[]  SumI2OutMax=[]  SumI3OutMin=[]  SumI3OutMax=[]  SumI4OutMin=[]  SumI4OutMax=[]  SumDOutMin=[]  SumDOutMax=[]  DifferentiatorOutMin=[]  DifferentiatorOutMax=[]  FilterDiffOutCoefMin=[]  FilterDiffOutCoefMax=[]  ReciprocalOutMin=[]  ReciprocalOutMax=[]  SumDenOutMin=[]  SumDenOutMax=[]  SumNumOutMin=[]  SumNumOutMax=[]  DivideOutMin=[]  DivideOutMax=[]  UdiffTsProdOutMin=[]  UdiffTsProdOutMax=[]  NTsProdOutMin=[]  NTsProdOutMax=[]  UintegralTsProdOutMin=[]  UintegralTsProdOutMax=[]  UngainTsProdOutMin=[]  UngainTsProdOutMax=[]  ClampingZeroOutDataTypeStr=Inherit: Inherit via back propagation  ClampingZeroOutMin=[]  ClampingZeroOutMax=[]  FilterDenConstantOutDataTypeStr=Inherit: Inherit via back propagation  FilterDenConstantOutMin=[]  FilterDenConstantOutMax=[]  PCopyOutDataTypeStr=Inherit: Inherit via back propagation  PCopyOutMin=[]  PCopyOutMax=[]  NCopyOutDataTypeStr=Inherit: Inherit via back propagation  NCopyOutMin=[]  NCopyOutMax=[]  IntegratorContinuousStateAttributes=''  IntegratorStateMustResolveToSignalObject=off  IntegratorRTWStateStorageClass=Auto  FilterContinuousStateAttributes=''  FilterStateMustResolveToSignalObject=off  FilterRTWStateStorageClass=Auto  ParallelPVariant=InternalParameters  IdealPVariant=Disabled  IVariant=InternalParameters  DVariant=Disabled  IntegratorVariant=Continuous  SatVariant=Disabled  AWVariant=Passthrough  PCopyVariant=Disabled  TRVariant=Disabled  FdbkBlocksVariant=Forward  IdealPFdbkVariant=Disabled  SatFdbkVariant=Disabled  DerivativeFilterVariant=Disabled  NVariant=Disabled  NCopyVariant=Disabled_SignalSpec  FilterICVariant=Disabled  IntegratorICVariant=InternalICs  ExternalResetVariant=Disabled  TRSumVariant=Passthrough  SumFdbkVariant=Disabled  SumVariant=Sum_PI  TsampFilterVariant=InternalTs  TsampNgainVariant=Passthrough  TsampIntegralVariant=Disabled_SignalSpec  ExternalSaturationOutDataTypeStr=Inherit: Same as second input
  Relational Operator : RelationalOperator  OutDataTypeStr=boolean  RndMeth=Simplest  InputSameDT=off
  Repeating Sequence : simulink/Sources/Repeating Sequence  rep_seq_t=[0, 1e-5, 2e-5]  rep_seq_y=[1, 0, 1]
  Scope : Scope
  Scope1 : Scope
  F : Outport
  wires:
  Relational Operator/1 -> F/1
  Repeating Sequence/1 -> Relational Operator/2
  Vref/1 -> Add/1
  Vmes/1 -> Add/2
  Add/1 -> PID Controller1/1, Scope/1
  PID Controller1/1 -> Scope1/1, Relational Operator/1

== system WindTurbine_System/SVPWM Rectifier/Space Vector PWM ==
  "Va, Vb, Vc" : Inport
  Add : Sum
  Add1 : Sum  Inputs=-+
  Gain : Gain  Gain=1.75/220
  Gain1 : Gain  Gain=0.5
  Gain2 : Gain  Gain=2/sqrt(3)
  MinMax1 : MinMax  InputSameDT=on  SaturateOnIntegerOverflow=on
  MinMax2 : MinMax  Function=max  InputSameDT=on  SaturateOnIntegerOverflow=on
  Relational Operator : RelationalOperator  Operator=>  InputSameDT=off
  Repeating Sequence : simulink/Sources/Repeating Sequence  rep_seq_t=[0 0.25 0.5 0.75 1]/10000  rep_seq_y=[1 0 -1 0 1]
  Scope{,1..3} (4 alike) : Scope
  Sa,Sb,Sc : Outport
  wires:
  "Va, Vb, Vc"/1 -> Gain/1
  Add/1 -> Gain1/1
  MinMax2/1 -> Add/2
  Gain2/1 -> Scope2/1, Relational Operator/1
  MinMax1/1 -> Add/1
  Gain/1 -> Scope3/1, MinMax1/1, MinMax2/1, Add1/2  "IGBT/Diode Voltage"
  Repeating Sequence/1 -> Relational Operator/2
  Gain1/1 -> Add1/1
  Add1/1 -> Scope/1, Gain2/1
  Relational Operator/1 -> Scope1/1, Sa,Sb,Sc/1

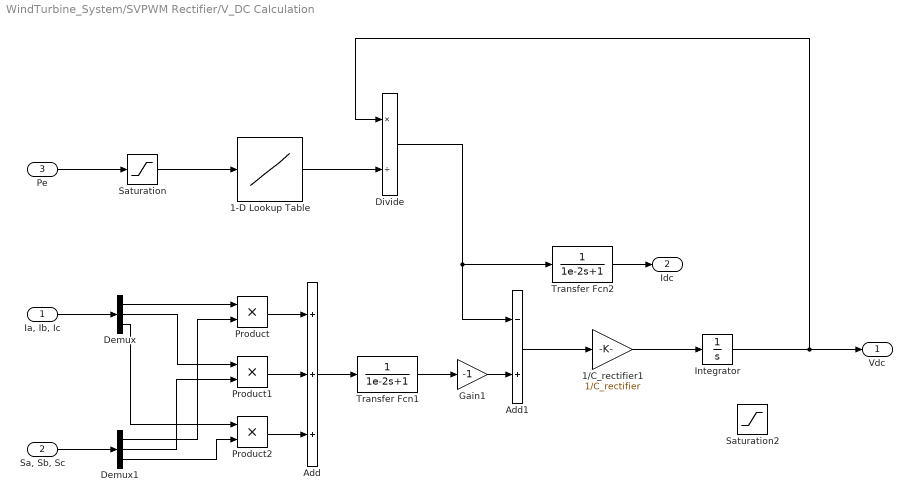
== system WindTurbine_System/SVPWM Rectifier/V_DC Calculation ==
  "Ia, Ib, Ic" : Inport
  "Sa, Sb, Sc" : Inport  Port=2
  Pe : Inport  Port=3
  1-D Lookup Table : Lookup_n-D  NumberOfTableDimensions=1  BreakpointsForDimension1=P_rec_v  Table=R_rec_load_v  InternalRulePriority=Speed  RndMeth=Simplest
  1/C_rectifier1 : Gain  Gain=1/C_rectifier
  Add : Sum  Inputs=+++
  Add1 : Sum  Inputs=-+
  Demux : Demux  Outputs=3
  Demux1 : Demux  Outputs=3
  Divide : Product  Inputs=*/
  Gain1 : Gain  Gain=-1
  Integrator : Integrator  UpperSaturationLimit=220  LowerSaturationLimit=-220
  Product : Product
  Product1 : Product
  Product2 : Product
  Saturation : Saturate  UpperLimit=inf  LowerLimit=1e-6
  Saturation2 : Saturate  UpperLimit=220  LowerLimit=-220
  Transfer Fcn1 : TransferFcn  Denominator=[1e-2 1]
  Transfer Fcn2 : TransferFcn  Denominator=[1e-2 1]
  Vdc : Outport
  Idc : Outport  Port=2
  wires:
  Product1/1 -> Add/2
  Demux/2 -> Product1/1
  Add/1 -> Transfer Fcn1/1
  Demux/1 -> Product/1
  Demux/3 -> Product2/1
  Product2/1 -> Add/3
  Demux1/1 -> Product/2
  Product/1 -> Add/1
  Demux1/2 -> Product1/2
  Add1/1 -> 1/C_rectifier1/1
  Demux1/3 -> Product2/2
  "Ia, Ib, Ic"/1 -> Demux/1
  "Sa, Sb, Sc"/1 -> Demux1/1
  Divide/1 -> Transfer Fcn2/1, Add1/1
  Transfer Fcn1/1 -> Gain1/1
  Pe/1 -> Saturation/1
  Saturation/1 -> 1-D Lookup Table/1
  1-D Lookup Table/1 -> Divide/2
  Gain1/1 -> Add1/2
  1/C_rectifier1/1 -> Integrator/1
  Integrator/1 -> Vdc/1, Divide/1
  Transfer Fcn2/1 -> Idc/1

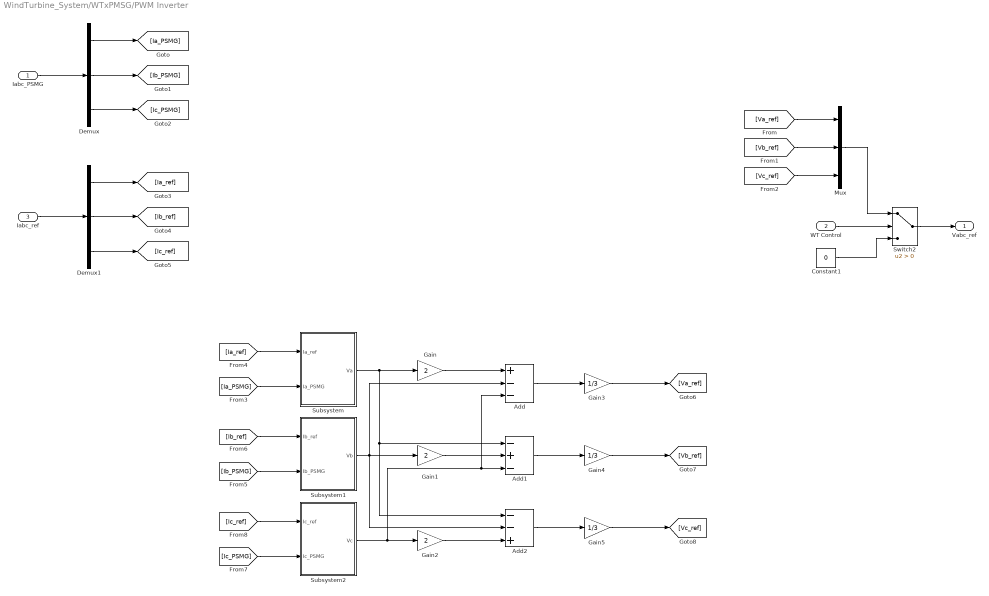
== system WindTurbine_System/WTxPMSG/PWM Inverter ==
  Iabc_PSMG : Inport
  WT Control : Inport  Port=2
  Iabc_ref : Inport  Port=3
  Add : Sum  Inputs=+--
  Add1 : Sum  Inputs=-+-
  Add2 : Sum  Inputs=--+
  Constant1 : Constant  Value=0
  Demux : Demux  Outputs=3
  Demux1 : Demux  Outputs=3
  Gain : Gain  Gain=2
  Gain1 : Gain  Gain=2
  Gain2 : Gain  Gain=2
  Gain3 : Gain  Gain=1/3
  Gain4 : Gain  Gain=1/3
  Gain5 : Gain  Gain=1/3
  Mux : Mux  Inputs=3
  Subsystem : Subsystem
  Subsystem1 : Subsystem
  Subsystem2 : Subsystem
  Switch2 : Switch  Criteria=u2 > Threshold  SaturateOnIntegerOverflow=off  InputSameDT=off
  Vabc_ref : Outport
  wires:
  Iabc_PSMG/1 -> Demux/1
  Demux/1 -> [Ia_PSMG]
  Demux/2 -> [Ib_PSMG]
  Demux/3 -> [Ic_PSMG]
  Demux1/3 -> [Ic_ref]
  Demux1/2 -> [Ib_ref]
  Demux1/1 -> [Ia_ref]
  Iabc_ref/1 -> Demux1/1
  [Va_ref] -> Mux/1
  [Vb_ref] -> Mux/2
  [Vc_ref] -> Mux/3
  [Ia_ref] -> Subsystem/1(Ia_ref)
  [Ia_PSMG] -> Subsystem/2(Ia_PSMG)
  [Ib_ref] -> Subsystem1/1(Ib_ref)
  [Ib_PSMG] -> Subsystem1/2(Ib_PSMG)
  [Ic_ref] -> Subsystem2/1(Ic_ref)
  [Ic_PSMG] -> Subsystem2/2(Ic_PSMG)
  Subsystem/1(Va) -> Add2/1, Add1/1, Gain/1
  Subsystem2/1(Vc) -> Add/3, Add1/3, Gain2/1
  Subsystem1/1(Vb) -> Add2/2, Gain1/1, Add/2
  Gain/1 -> Add/1
  Gain1/1 -> Add1/2
  Gain2/1 -> Add2/3
  Add/1 -> Gain3/1
  Add1/1 -> Gain4/1
  Add2/1 -> Gain5/1
  Gain5/1 -> [Vc_ref]
  Gain4/1 -> [Vb_ref]
  Gain3/1 -> [Va_ref]
  Constant1/1 -> Switch2/3
  WT Control/1 -> Switch2/2
  Switch2/1 -> Vabc_ref/1
  Mux/1 -> Switch2/1

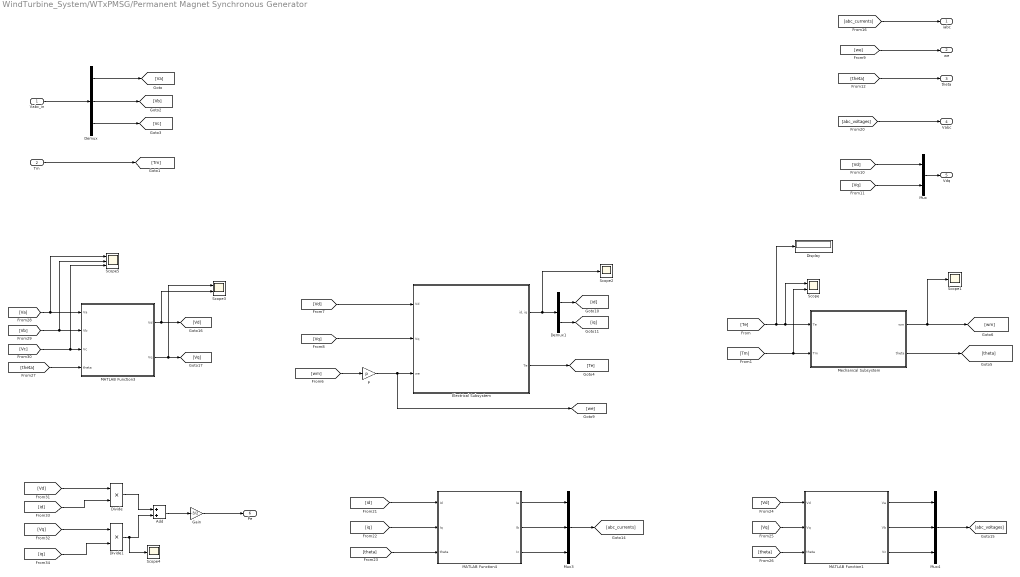
== system WindTurbine_System/WTxPMSG/Permanent Magnet Synchronous Generator ==
  Vabc_in : Inport
  Tm : Inport  Port=2
  Add : Sum
  Demux : Demux  Outputs=3
  Demux1 : Demux  Outputs=2
  Display : Display
  Divide : Product  Inputs=**
  Divide1 : Product  Inputs=**
  Electrical Subsystem : Subsystem
  Gain : Gain  Gain=-3/2
  MATLAB Function1 : MATLAB Function  TreatAsAtomicUnit=on
  MATLAB Function3 : MATLAB Function  TreatAsAtomicUnit=on
  MATLAB Function4 : MATLAB Function  TreatAsAtomicUnit=on
  Mechanical Subsystem : Subsystem
  Mux : Mux  Inputs=2
  Mux3 : Mux  Inputs=3
  Mux4 : Mux  Inputs=3
  P : Gain  Gain=p
  Scope : Scope  NumInputPorts=2
  Scope1 : Scope
  Scope2 : Scope
  Scope3 : Scope  NumInputPorts=2
  Scope4 : Scope
  Scope5 : Scope  NumInputPorts=3
  iabc : Outport
  we : Outport  Port=2
  theta : Outport  Port=3
  Vabc : Outport  Port=4
  Vdq : Outport  Port=5
  Pe : Outport  Port=6
  wires:
  Vabc_in/1 -> Demux/1
  Tm/1 -> [Tm]
  Demux/1 -> [Va]
  Demux/2 -> [Vb]
  Demux/3 -> [Vc]
  Electrical Subsystem/2(Te) -> [Te]
  [Te] -> Display/1, Scope/1, Mechanical Subsystem/1(Te)
  [Tm] -> Scope/2, Mechanical Subsystem/2(Tm)
  Mechanical Subsystem/1(wm) -> Scope1/1, [wm]
  [wm] -> P/1
  P/1 -> [we], Electrical Subsystem/3(we)
  [Vq] -> Electrical Subsystem/2(Vq)
  [Vd] -> Electrical Subsystem/1(Vd)
  [we] -> we/1
  Mux/1 -> Vdq/1
  [Vd] -> Mux/1
  [Vq] -> Mux/2
  [theta] -> theta/1
  Electrical Subsystem/1("id, iq") -> Scope2/1, Demux1/1
  Demux1/1 -> [id]
  Demux1/2 -> [iq]
  [abc_currents] -> iabc/1
  [abc_voltages] -> Vabc/1
  [iq] -> MATLAB Function4/2(Iq)
  [theta] -> MATLAB Function4/3(theta)
  [id] -> MATLAB Function4/1(Id)
  Mux3/1 -> [abc_currents]
  MATLAB Function4/2(Ib) -> Mux3/2
  MATLAB Function4/1(Ia) -> Mux3/1
  MATLAB Function4/3(Ic) -> Mux3/3
  [Vd] -> MATLAB Function1/1(Vd)
  [Vq] -> MATLAB Function1/2(Vq)
  [theta] -> MATLAB Function1/3(theta)
  Mux4/1 -> [abc_voltages]
  MATLAB Function1/1(Va) -> Mux4/1
  MATLAB Function1/2(Vb) -> Mux4/2
  MATLAB Function1/3(Vc) -> Mux4/3
  [Va] -> Scope5/1, MATLAB Function3/1(Va)
  [Vc] -> Scope5/3, MATLAB Function3/3(Vc)
  [theta] -> MATLAB Function3/4(theta)
  [Vb] -> Scope5/2, MATLAB Function3/2(Vb)
  MATLAB Function3/2(Vq) -> Scope3/1, [Vq]
  MATLAB Function3/1(Vd) -> Scope3/2, [Vd]
  [Vq] -> Divide1/1
  [iq] -> Divide1/2
  [id] -> Divide/2
  [Vd] -> Divide/1
  Divide/1 -> Add/1
  Divide1/1 -> Scope4/1, Add/2
  Add/1 -> Gain/1
  Gain/1 -> Pe/1
  Mechanical Subsystem/2(theta) -> [theta]

== system WindTurbine_System/WTxPMSG/Subsystem ==
  Unfiltered Vabc : Inport
  Demux : Demux  Outputs=3
  Mux1 : Mux  Inputs=3
  Transfer Fcn1 : TransferFcn  Denominator=[1e-4 1]
  Transfer Fcn2 : TransferFcn  Denominator=[1e-4 1]
  Transfer Fcn3 : TransferFcn  Denominator=[1e-4 1]
  Filtered Vabc : Outport
  wires:
  Unfiltered Vabc/1 -> Demux/1
  Mux1/1 -> Filtered Vabc/1
  Transfer Fcn2/1 -> Mux1/2
  Transfer Fcn1/1 -> Mux1/1
  Demux/1 -> Transfer Fcn1/1
  Demux/2 -> Transfer Fcn2/1
  Transfer Fcn3/1 -> Mux1/3
  Demux/3 -> Transfer Fcn3/1

== system WindTurbine_System/WTxPMSG/Subsystem1 ==
  Unfiltered Power : Inport
  Saturation : Saturate  UpperLimit=4500  LowerLimit=-45
  Transfer Fcn : TransferFcn  Denominator=[1e-2 1]
  Filtered Power : Outport
  wires:
  Transfer Fcn/1 -> Saturation/1
  Unfiltered Power/1 -> Transfer Fcn/1
  Saturation/1 -> Filtered Power/1

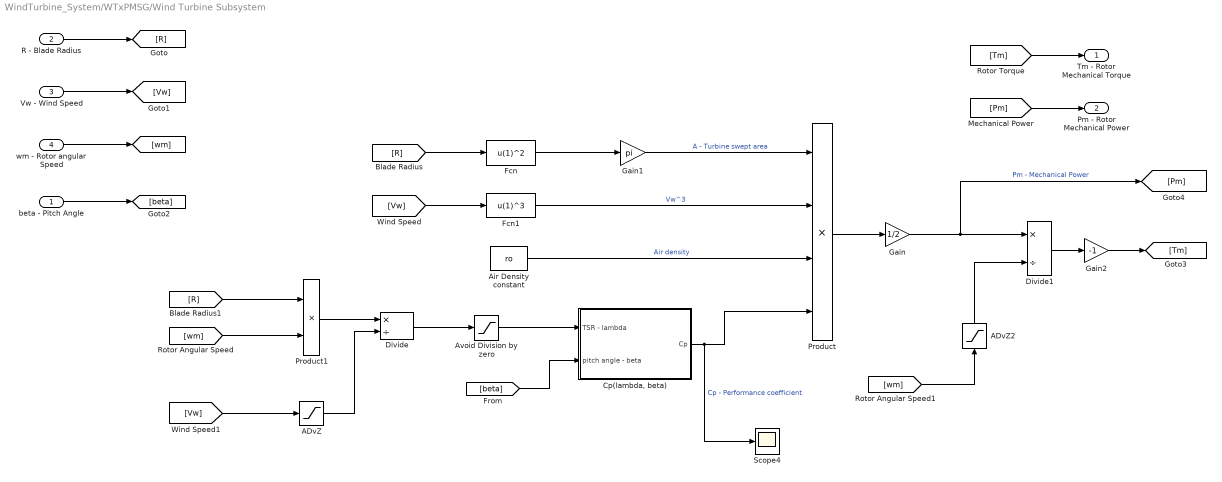
== system WindTurbine_System/WTxPMSG/Wind Turbine Subsystem ==
  beta - Pitch Angle : Inport
  R - Blade Radius : Inport  Port=2
  Vw - Wind Speed : Inport  Port=3
  wm - Rotor angular Speed : Inport  Port=4
  ADvZ : Saturate  UpperLimit=1e6  LowerLimit=1e-6
  ADvZ2 : Saturate  UpperLimit=omega_r  LowerLimit=1e-6
  Air Density constant : Constant  Value=ro
  Avoid Division by zero : Saturate  UpperLimit=Inf  LowerLimit=1e-6
  "Cp(lambda, beta)" : Subsystem
  Divide : Product  Inputs=*/
  Divide1 : Product  Inputs=*/
  Fcn : Fcn  Expr=u(1)^2
  Fcn1 : Fcn  Expr=u(1)^3
  Gain : Gain  Gain=1/2
  Gain1 : Gain  Gain=pi
  Gain2 : Gain  Gain=-1
  Product : Product  Inputs=4
  Product1 : Product
  Scope4 : Scope
  Tm - Rotor Mechanical Torque : Outport
  Pm - Rotor Mechanical Power : Outport  Port=2
  wires:
  Product/1 -> Gain/1
  Gain1/1 -> Product/1  "A - Turbine swept area"
  Fcn1/1 -> Product/2  "Vw^3"
  Air Density constant/1 -> Product/3  "Air density"
  "Cp(lambda, beta)"/1(Cp) -> Scope4/1, Product/4  "Cp - Performance coefficient"
  Fcn/1 -> Gain1/1
  R - Blade Radius/1 -> [R]
  Vw - Wind Speed/1 -> [Vw]
  [R] -> Fcn/1
  [Vw] -> Fcn1/1
  wm - Rotor angular Speed/1 -> [wm]
  [R] -> Product1/1
  [wm] -> Product1/2
  Product1/1 -> Divide/1
  [Vw] -> ADvZ/1
  Divide/1 -> Avoid Division by zero/1
  ADvZ/1 -> Divide/2
  beta - Pitch Angle/1 -> [beta]
  [beta] -> "Cp(lambda, beta)"/2(pitch angle - beta)
  [Tm] -> Tm - Rotor Mechanical Torque/1
  Gain/1 -> Divide1/1, [Pm]  "Pm - Mechanical Power"
  Divide1/1 -> Gain2/1
  [wm] -> ADvZ2/1
  [Pm] -> Pm - Rotor Mechanical Power/1
  ADvZ2/1 -> Divide1/2
  Avoid Division by zero/1 -> "Cp(lambda, beta)"/1(TSR - lambda)
  Gain2/1 -> [Tm]

== system WindTurbine_System/WTxPMSG/PWM Inverter/Subsystem ==
  Ia_ref : Inport
  Ia_PSMG : Inport  Port=2
  Add : Sum  Inputs=+-
  Filtru curent : TransferFcn  Denominator=[5e-6 1]
  Relay : Relay  OnSwitchValue=0.05  OffSwitchValue=-0.05  OnOutputValue=155  OffOutputValue=-155
  Scope : Scope  NumInputPorts=2
  Scope1 : Scope  NumInputPorts=2
  Scope2 : Scope
  Va : Outport
  wires:
  Ia_ref/1 -> Scope/1, Add/1
  Ia_PSMG/1 -> Scope1/1, Filtru curent/1
  Filtru curent/1 -> Scope1/2, Scope/2, Add/2
  Add/1 -> Relay/1
  Relay/1 -> Scope2/1, Va/1

== system WindTurbine_System/WTxPMSG/PWM Inverter/Subsystem1 ==
  Ib_ref : Inport
  Ib_PSMG : Inport  Port=2
  Add : Sum  Inputs=+-
  Filtru curent : TransferFcn  Denominator=[5e-6 1]
  Relay : Relay  OnSwitchValue=0.05  OffSwitchValue=-0.05  OnOutputValue=155  OffOutputValue=-155
  Vb : Outport
  wires:
  Relay/1 -> Vb/1
  Add/1 -> Relay/1
  Filtru curent/1 -> Add/2
  Ib_PSMG/1 -> Filtru curent/1
  Ib_ref/1 -> Add/1

== system WindTurbine_System/WTxPMSG/PWM Inverter/Subsystem2 ==
  Ic_ref : Inport
  Ic_PSMG : Inport  Port=2
  Add : Sum  Inputs=+-
  Filtru curent : TransferFcn  Denominator=[5e-6 1]
  Relay : Relay  OnSwitchValue=0.05  OffSwitchValue=-0.05  OnOutputValue=155  OffOutputValue=-155
  Vc : Outport
  wires:
  Ic_ref/1 -> Add/1
  Ic_PSMG/1 -> Filtru curent/1
  Filtru curent/1 -> Add/2
  Add/1 -> Relay/1
  Relay/1 -> Vc/1

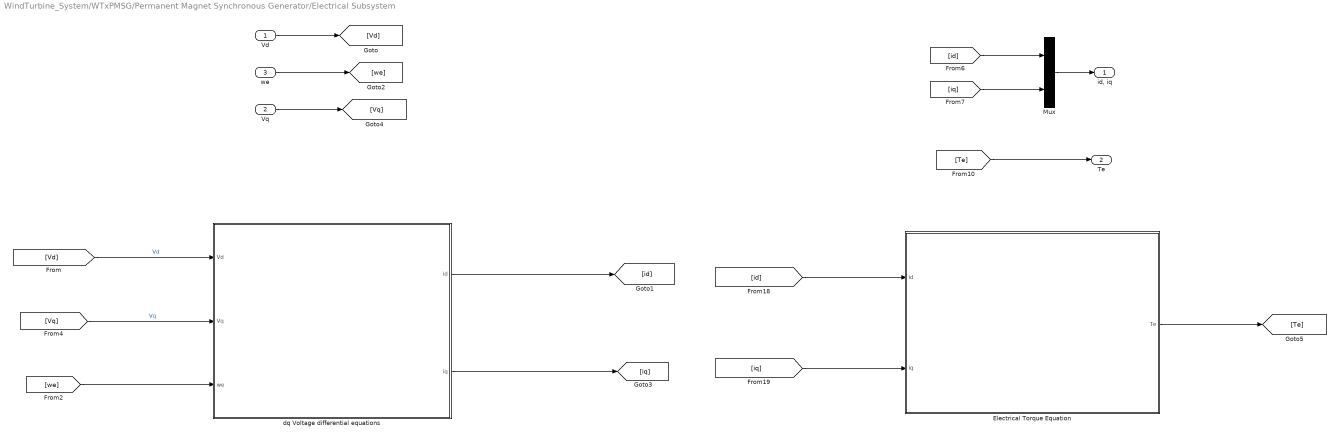
== system WindTurbine_System/WTxPMSG/Permanent Magnet Synchronous Generator/Electrical Subsystem ==
  Vd : Inport
  Vq : Inport  Port=2
  we : Inport  Port=3
  Electrical Torque Equation : Subsystem
  Mux : Mux  Inputs=2
  dq Voltage differential equations : Subsystem
  "id, iq" : Outport
  Te : Outport  Port=2
  wires:
  Vd/1 -> [Vd]
  we/1 -> [we]
  Vq/1 -> [Vq]
  Mux/1 -> "id, iq"/1
  [id] -> Mux/1
  [iq] -> Mux/2
  [Te] -> Te/1
  [Vd] -> dq Voltage differential equations/1(Vd)  "Vd"
  [Vq] -> dq Voltage differential equations/2(Vq)  "Vq"
  dq Voltage differential equations/1(id) -> [id]
  dq Voltage differential equations/2(iq) -> [iq]
  [id] -> Electrical Torque Equation/1(id)
  [iq] -> Electrical Torque Equation/2(iq)
  Electrical Torque Equation/1(Te) -> [Te]
  [we] -> dq Voltage differential equations/3(we)

== system WindTurbine_System/WTxPMSG/Permanent Magnet Synchronous Generator/Mechanical Subsystem ==
  Te : Inport
  Tm : Inport  Port=2
  Divide : Product  Inputs=*/
  Frecare vascoasa : Gain  Gain=1e-3
  Integrator : Integrator
  Integrator1 : Integrator
  J : Constant  Value=J
  Scope : Scope
  Subtract : Sum  Inputs=+--
  wm : Outport
  theta : Outport  Port=2
  wires:
  Te/1 -> Subtract/1
  Subtract/1 -> Scope/1, Divide/1
  J/1 -> Divide/2
  Divide/1 -> Integrator/1  "(Te-Tm)/J"
  Integrator/1 -> Frecare vascoasa/1, Integrator1/1, wm/1  "wm"
  Integrator1/1 -> theta/1  "theta"
  Frecare vascoasa/1 -> Subtract/3
  Tm/1 -> Subtract/2

== system WindTurbine_System/WTxPMSG/Wind Turbine Subsystem/Cp(lambda, beta) ==
  TSR - lambda : Inport
  pitch angle - beta : Inport  Port=2
  1/lambda_i equation : Fcn  Expr=1/(u(1)+0.08*u(2)) - 0.035/(1+u(2)^3)
  "Cp(lambda, beta) equation" : Fcn  Expr=c1*(c2*u(1) - c3*u(2) - c5)*exp(-c6*u(1))
  Mux : Mux  Inputs=2
  Mux1 : Mux  Inputs=2
  Cp : Outport
  wires:
  "Cp(lambda, beta) equation"/1 -> Cp/1
  Mux/1 -> "Cp(lambda, beta) equation"/1
  1/lambda_i equation/1 -> Mux/1  "u(1)"
  pitch angle - beta/1 -> Mux/2, Mux1/2  "u(2)"
  Mux1/1 -> 1/lambda_i equation/1
  TSR - lambda/1 -> Mux1/1  "u(1)"

== system WindTurbine_System/WTxPMSG/Permanent Magnet Synchronous Generator/Electrical Subsystem/Electrical Torque Equation ==
  id : Inport
  iq : Inport  Port=2
  " " : Gain  Gain=3/2
  Add2 : Sum
  Divide5 : Product  Inputs=**
  Divide6 : Product  Inputs=***
  Divide7 : Product  Inputs=**
  Ke : Constant  Value=Ke
  Ld : Constant  Value=Ld
  Lq2 : Constant  Value=Lq
  Subtract : Sum  Inputs=+-
  p : Constant  Value=p
  Te : Outport
  wires:
  id/1 -> Divide6/2
  [Ke] -> Divide7/2
  Divide5/1 -> Te/1  "Te"
  " "/1 -> Divide5/2
  iq/1 -> Divide7/1, Divide6/3
  [Ld] -> Subtract/1
  Subtract/1 -> Divide6/1
  p/1 -> " "/1
  Add2/1 -> Divide5/1
  Divide6/1 -> Add2/1  "(Ld-Lq)*id*iq"
  [Lq] -> Subtract/2
  Divide7/1 -> Add2/2  "Ke*iq"
  Ld/1 -> [Ld]
  Lq2/1 -> [Lq]
  Ke/1 -> [Ke]

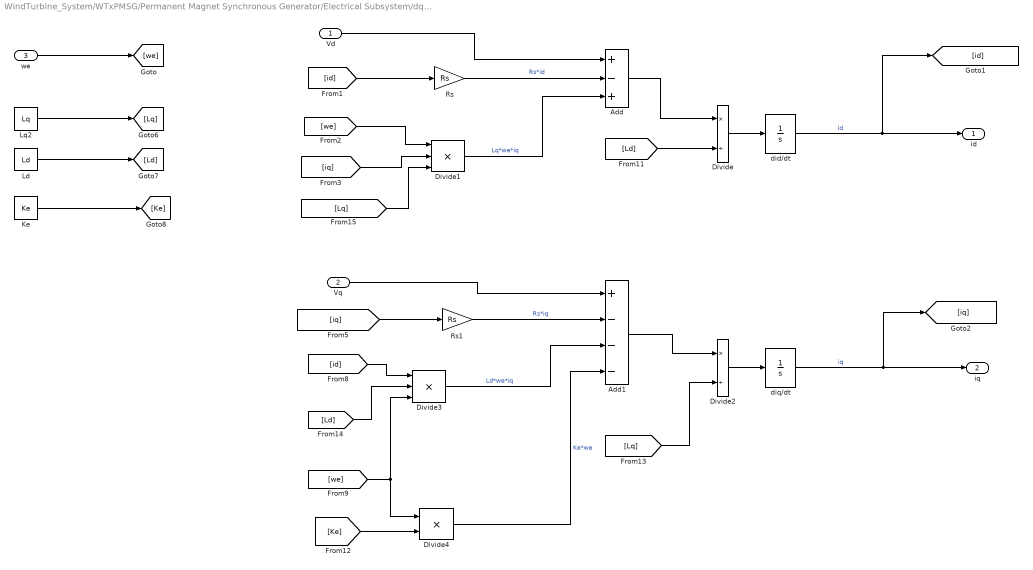
== system WindTurbine_System/WTxPMSG/Permanent Magnet Synchronous Generator/Electrical Subsystem/dq Voltage differential equations ==
  Vd : Inport
  Vq : Inport  Port=2
  we : Inport  Port=3
  Add : Sum  Inputs=+-+
  Add1 : Sum  Inputs=+---
  Divide : Product  Inputs=*/
  Divide1 : Product  Inputs=***
  Divide2 : Product  Inputs=*/
  Divide3 : Product  Inputs=***
  Divide4 : Product  Inputs=**
  Ke : Constant  Value=Ke
  Ld : Constant  Value=Ld
  Lq2 : Constant  Value=Lq
  Rs : Gain  Gain=Rs
  Rs1 : Gain  Gain=Rs
  did/dt : Integrator
  diq/dt : Integrator
  id : Outport
  iq : Outport  Port=2
  wires:
  diq/dt/1 -> [iq], iq/1  "iq"
  Add/1 -> Divide/1
  did/dt/1 -> [id], id/1  "id"
  Rs1/1 -> Add1/2  "Rs*iq"
  [Lq] -> Divide2/2
  Vq/1 -> Add1/1
  [iq] -> Divide1/2
  [id] -> Divide3/1
  Divide1/1 -> Add/3  "Lq*we*iq"
  Add1/1 -> Divide2/1
  [iq] -> Rs1/1
  [Ld] -> Divide3/2
  Divide2/1 -> diq/dt/1
  [Lq] -> Divide1/3
  Rs/1 -> Add/2  "Rs*id"
  [we] -> Divide1/1
  Divide/1 -> did/dt/1
  [Ke] -> Divide4/2
  [we] -> Divide3/3, Divide4/1
  Divide4/1 -> Add1/4  "Ke*we"
  Divide3/1 -> Add1/3  "Ld*we*iq"
  [id] -> Rs/1
  Vd/1 -> Add/1
  [Ld] -> Divide/2
  Ld/1 -> [Ld]
  Lq2/1 -> [Lq]
  Ke/1 -> [Ke]
  we/1 -> [we]

== matlab function WindTurbine_System/MATLAB Function ==
  settings: updateMethod=DISCRETE
  data: simTime input; cost output; hour input; Energy_Deficit input
function cost = Cost_Func(simTime, hour, Energy_Deficit)

    persistent total_cost last_hour deficit_start_time deficit_active deficit_sum deficit_count;

    if isempty(total_cost)
        total_cost = 0;
        last_hour = -1;
        deficit_start_time = 0;
        deficit_active = false;
        deficit_sum = 0;
        deficit_count = 0;
    end

    % Verificam daca suntem intr-un nou ciclu de ora

    if hour ~= last_hour

        % Daca exista deficit se calculeaza si adauga deficitul din ora
        % precedenta

        if deficit_active

            rate = getRate(last_hour);
            hourly_cost = calculateHourlyCost(rate, deficit_start_time, simTime, deficit_sum / deficit_count);
            total_cost = total_cost + hourly_cost;
            deficit_active = false;  

        end

        last_hour = hour;
        deficit_sum = 0;  
        deficit_count = 0;

    end

    % Verificăm dacă există un deficit de energie
    if Energy_Deficit < 0

        if ~deficit_active
            deficit_start_time = simTime;
            deficit_active = true;
        end

        deficit_sum = deficit_sum + Energy_Deficit;
        deficit_count = deficit_count + 1;

    elseif deficit_active

        % Calculează și adaugă costul pentru perioada de deficit
        rate = getRate(last_hour);
        hourly_cost = calculateHourlyCost(rate, deficit_start_time, simTime, deficit_sum / deficit_count);
        total_cost = total_cost + hourly_cost;
        deficit_active = false;

    end

    cost = total_cost;

end

function rate = getRate(hour)

    if hour >= 10 && hour < 18
        rate = 1.13;
    else
        rate = 0.8;
    end

end

function h_cost = calculateHourlyCost(rate, start_time, end_time, deficit)

    h_cost = (end_time - start_time) * (-deficit) * rate / 1000;

end
